simulink model "task_D_mod"  (R2018a)
settings: Solver=ode4  StartTime=0.0  StopTime=10.0  FixedStep=0.01  RelTol=1e-3  EnableMultiTasking=on
values from neighbouring files (symbols this model uses):
  a0 = 2    [task_D_scr.m]    (also in task_E_scr.m; task_F_scr.m)
  b = 2*n*sqrt(p^2-n^2)    [task_B_scr.m]    (also in task_C_scr.m; task_D_scr.m; task_E_scr.m; task_F_scr.m)
  b0 = 1    [task_D_scr.m]    (also in task_E_scr.m; task_F_scr.m)
  Ln = 1; sim('task_A_mod')    [task_A_scr.m]    (also in task_C_scr.m = 10; sim('task_C_mod'); task_D_scr.m = 10; sim('task_D_mod'); task_E_scr.m = 10; sim('task_E_mod',5); task_F_scr.m = 10; sim('task_E_mod',20))
  n = 10    [task_B_scr.m]    (also in task_C_scr.m = 8; task_D_scr.m; task_E_scr.m; task_F_scr.m)
  p = sqrt(W^2+2*n^2)    [task_B_scr.m]    (also in task_C_scr.m = sqrt(1+2*n^2); task_D_scr.m = sqrt(2*n^2); task_E_scr.m = sqrt(2*n^2); task_F_scr.m = sqrt(2*n^2))
settings Model: Creator=Yurii  LastModifiedBy=Master
settings DataIOCC: LimitDataPoints=on  SaveFormat=Array
settings OptimizationCC: LifeSpan=inf
settings DebuggingCC: UnderspecifiedInitializationDetection=Classic  MergeDetectMultiDrivingBlocksExec=none  SolverPrmCheckMsg=warning  SFUnexpectedBacktrackingDiag=warning  SFNoUnconditionalDefaultTransitionDiag=warning  SFExecutionAtInitializationDiag=none
settings HardwareCC: ProdBitPerPointer=32  ProdBitPerSizeT=32  ProdBitPerPtrDiffT=32  ProdLargestAtomicFloat=None  ProdIntDivRoundTo=Undefined  ProdEndianess=Unspecified  ProdWordSize=32  ProdHWDeviceType=32-bit Generic
settings ModelReferenceCC: PropagateSignalLabelsOutOfModel=off
settings CodeAppCC: StateflowObjectComments=on
settings GRTTargetCC: TargetLangStandard=C89/C90 (ANSI)  GeneratePreprocessorConditionals=Disable all
settings ConfigComp: CovMetricSettings=dw  CovHtmlReporting=on  CovSaveCumulativeToWorkspaceVar=on  CovSaveSingleToWorkspaceVar=on  CovExternalEMLEnable=off

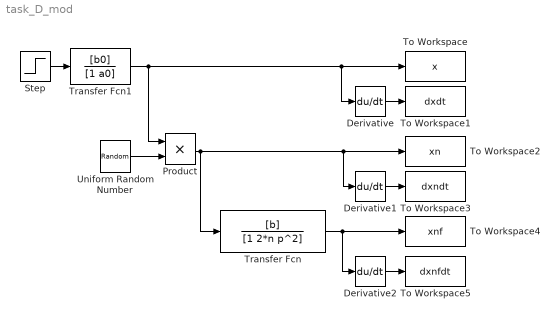
== system task_D_mod ==
  Derivative : Derivative
  Derivative1 : Derivative
  Derivative2 : Derivative
  Product : Product
  Step : Step  SampleTime=0
  To Workspace : ToWorkspace  VariableName=x  SaveFormat=Timeseries  SampleTime=-1
  To Workspace1 : ToWorkspace  VariableName=dxdt  SaveFormat=Timeseries  SampleTime=-1
  To Workspace2 : ToWorkspace  VariableName=xn  SaveFormat=Timeseries  SampleTime=-1
  To Workspace3 : ToWorkspace  VariableName=dxndt  SaveFormat=Timeseries  SampleTime=-1
  To Workspace4 : ToWorkspace  VariableName=xnf  SaveFormat=Timeseries  SampleTime=-1
  To Workspace5 : ToWorkspace  VariableName=dxnfdt  SaveFormat=Timeseries  SampleTime=-1
  Transfer Fcn : TransferFcn  Numerator=[b]  Denominator=[1 2*n p^2]
  Transfer Fcn1 : TransferFcn  Numerator=[b0]  Denominator=[1 a0]
  Uniform Random Number : UniformRandomNumber  Minimum=1-Ln/100  Maximum=1+Ln/100  SampleTime=0.0
  wires:
  Transfer Fcn1/1 -> Product/1, Derivative/1, To Workspace/1
  Derivative/1 -> To Workspace1/1
  Uniform Random Number/1 -> Product/2
  Product/1 -> Transfer Fcn/1, Derivative1/1, To Workspace2/1
  Derivative1/1 -> To Workspace3/1
  Transfer Fcn/1 -> Derivative2/1, To Workspace4/1
  Derivative2/1 -> To Workspace5/1
  Step/1 -> Transfer Fcn1/1
